simulink library "aerolibadyn"  (Simulink 5.0)
libraries: aerolibbdyn x1
settings Model: Creator=sgage  LastModifiedBy=sgage  ExtModeAutoUpdateStatusClock=off  TargetHWChar=2  TargetHWWordLengths=8,16,32,32

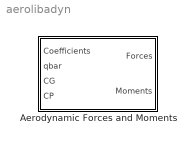
== system aerolibadyn ==
  Aerodynamic Forces and Moments : Subsystem  mask(Aerodynamic Forces and Moments){S=1, b=1, cbar=1}
      mask prompts: S "Reference area:"; b "Reference span:"; cbar "Reference length:"
      mask help: Compute the aerodynamic forces and moments applied at the center of gravity using the aerodynamic coefficients, dynamic pressure, center of gravity and center of pressure.
      mask Help: web(asbhelp);
      mask Display:
      | port_label('input',1,'Coefficients','texmode','on');
      | port_label('input',2,'q_{bar}','texmode','on');
      | port_label('input',3,'CG','texmode','on');
      | port_label('input',4,'CP','texmode','on');
      | port_label('output',1,'F_{aero}','texmode','on');
      | port_label('output',2,'M_{aero}','texmode','on');

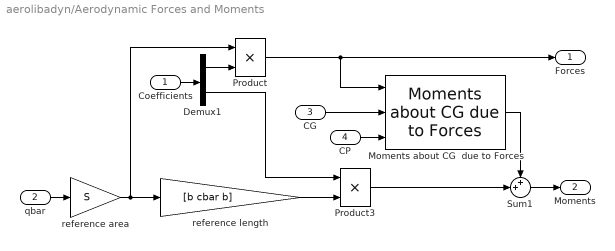
== system aerolibadyn/Aerodynamic Forces and Moments ==
  Coefficients : Inport
  qbar : Inport  Port=2
  CG : Inport  Port=3
  CP : Inport  Port=4
  Demux1 : Demux  Outputs=[3,3]
  Moments about CG  due to Forces : aerolibbdyn/Moments about CG  due to Forces
  Product : Product  SaturateOnIntegerOverflow=on  InputSameDT=on
  Product3 : Product  SaturateOnIntegerOverflow=on  InputSameDT=on
  Sum1 : Sum  Inputs=++|  SaturateOnIntegerOverflow=on  InputSameDT=on
  reference area : Gain  Gain=S  SaturateOnIntegerOverflow=on
  reference length : Gain  Gain=[b cbar b]  SaturateOnIntegerOverflow=on
  Forces : Outport
  Moments : Outport  Port=2
  wires:
  CP/1 -> Moments about CG  due to Forces/3
  CG/1 -> Moments about CG  due to Forces/2
  Sum1/1 -> Moments/1
  Product3/1 -> Sum1/2
  Product/1 -> Forces/1, Moments about CG  due to Forces/1
  reference area/1 -> Product/1, reference length/1
  qbar/1 -> reference area/1
  Demux1/2 -> Product3/1
  Demux1/1 -> Product/2
  Coefficients/1 -> Demux1/1
  reference length/1 -> Product3/2
  Moments about CG  due to Forces/1 -> Sum1/1
